simulink model "DQGEN"  (R2023b)
settings: Solver=ode23tb  StartTime=0.0  StopTime=0.1  FixedStep=Ts  RelTol=1e-5  EnableMultiTasking=on
values from neighbouring files (symbols this model uses):
  N = 2    [DQGEN_calc.m]
  Ts = 50e-6    (= 5e-05)    [DQGEN_calc.m]
  Ts_dqn = Ts    (= 5e-05)    [DQGEN_calc.m]
  Ws = 2*pi*f    (= 376.991118431)    [DQGEN_calc.m]
undefined symbols (not defined in the file or in its folder): DiscIntNeverNeededParam, rlc, SYS
libraries: spsThreePhaseVIMeasurementLib x3, DQN_Lib x2, spsLoadFlowBusLib x2, spsMultimeterLib x2, spsSteamTurbineandGovernorLib x2, spsThreePhaseSourceLib x1, spsGroundLib x1, spsSynchronousMachinepuStandardLib x1, spsThreePhaseParallelRLCBranchLib x1, spsThreePhaseSeriesRLCBranchLib x1, spsabctodq0Lib x1, spspowerguiLib x1
(part 1 of 2)
settings Model: NumberOfSteps=10  PacingRate=0.005000  Creator=The MathWorks, Inc.  LastModifiedBy=rober
settings SolverCC: ZeroCrossControl=DisableAll  ZeroCrossAlgorithm=Adaptive  AlgebraicLoopSolver=TrustRegion
settings DataIOCC: SaveFormat=Array  SaveOutput=off  SaveTime=off  ReturnWorkspaceOutputs=off  TimeSaveName=t  SignalLoggingName=sigsOut
settings OptimizationCC: BlockReduction=off  BooleanDataType=off  ExpressionDepthLimit=2147483647  InitFltsAndDblsToZero=on  EfficientMapNaN2IntZero=off  LifeSpan=inf
settings DebuggingCC: UnderspecifiedInitializationDetection=Classic  MergeDetectMultiDrivingBlocksExec=none  CheckExecutionContextPreStartOutputMsg=on  SignalResolutionControl=TryResolveAllWithWarning  IgnoredZcDiagnostic=none  MultiTaskDSMMsg=warning  MultiTaskCondExecSysMsg=none  FcnCallInpInsideContextMsg=warning  StateNameClashWarn=warning  SFUnexpectedBacktrackingDiag=warning  SFNoUnconditionalDefaultTransitionDiag=warning  SFExecutionAtInitializationDiag=none  ArithmeticOperatorsInVariantConditions=warning
settings HardwareCC: ProdBitPerPointer=32  ProdBitPerSizeT=32  ProdBitPerPtrDiffT=32  ProdLargestAtomicFloat=None  ProdIntDivRoundTo=Undefined  ProdEndianess=Unspecified  ProdWordSize=32  ProdHWDeviceType=32-bit Generic  TargetBitPerPointer=64  TargetBitPerSizeT=64  TargetBitPerPtrDiffT=64  TargetLongLongMode=on  TargetIntDivRoundTo=Zero  TargetEndianess=LittleEndian  TargetWordSize=64  TargetHWDeviceType=MATLAB Host  ProdEqTarget=off
settings ModelReferenceCC: EnableRefExpFcnMdlSchedulingChecks=on  PropagateSignalLabelsOutOfModel=off
settings SFSimCC: SimUseLocalCustomCode=off  CustomCodeUndefinedFunction=UseInterfaceOnly
settings RTWCC: RTWUseLocalCustomCode=off  DLArmComputeVersion=19.05
settings CodeAppCC: StateflowObjectComments=on
settings GRTTargetCC: TargetLangStandard=C89/C90 (ANSI)  CombineOutputUpdateFcns=off  GRTInterface=on
settings ConfigComp: CovMetricSettings=dw  CovSaveCumulativeToWorkspaceVar=on  CovSaveSingleToWorkspaceVar=on  CovExternalEMLEnable=off  CovSFcnEnable=off
settings SimscapeCC: SimscapeNormalizeSystem=off

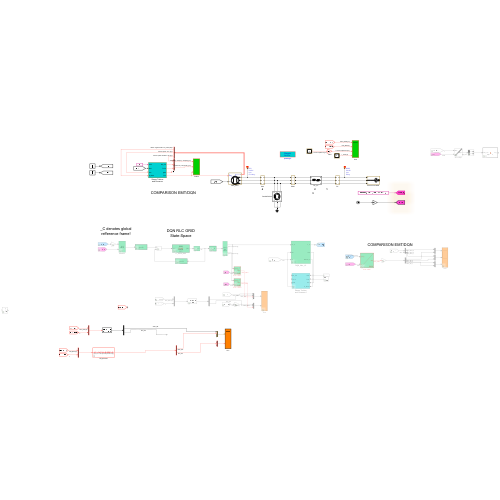
[thumbnail: Simulink's stored preview of the top-level diagram]
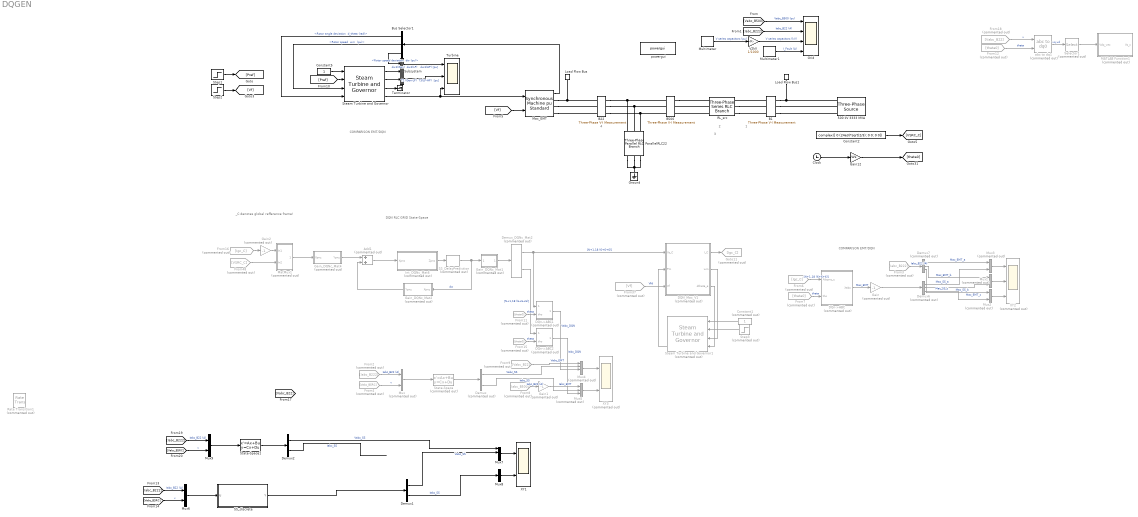
== system DQGEN ==
  note: DQN RLC GRID
      | State-Space
  note: 1
  note: 2
  note: 3
  note: 4
  note: COMPARISON EMT/DQN
  note: _C denotes global
      | refference frame!
  note: COMPARISON EMT/DQN
  500 kV 3333 MVA : spsThreePhaseSourceLib/Three-Phase Source  InternalConnection=Yg  VoltagePhases=off  Voltage=(24000)*1  PhaseAngle=0  Voltage_phases=[25e3 25e3 25e3]/sqrt(3)  PhaseAngles_phases=[0 -120 +120]  Frequency=60  NonIdealSource=off  SpecifyImpedance=on  Resistance=3.5  Inductance=0.1989  ShortCircuitLevel=3333e6  BaseVoltage=500e3  XRratio=21.43  BusType=swing  Pref=0  Qref=0  Prefabc=[10e3, 10e3, 10e3]  Qrefabc=[0, 0, 0]  Qmin=-Inf  Qmax=Inf
  Add1 : Sum  Commented=on
  B1 : spsThreePhaseVIMeasurementLib/Three-Phase V-I Measurement  VoltageMeasurement=phase-to-ground  SetLabelV=on  LabelV=Vabc_BSRC  Vpu=off  VpuLL=off  CurrentMeasurement=yes  SetLabelI=on  LabelI=Iabc_BSRC  Ipu=off  Pbase=100e6  Vbase=500e3  OutputType=Complex  PhasorSimulation=off  PSBequivalent=0
  B22 : spsThreePhaseVIMeasurementLib/Three-Phase V-I Measurement  VoltageMeasurement=phase-to-ground  SetLabelV=on  LabelV=Vabc_B22  Vpu=off  VpuLL=off  CurrentMeasurement=yes  SetLabelI=on  LabelI=Iabc_B222  Ipu=off  Pbase=555e6  Vbase=24e3  OutputType=Complex  PhasorSimulation=off  PSBequivalent=0
  B500 : spsThreePhaseVIMeasurementLib/Three-Phase V-I Measurement  VoltageMeasurement=phase-to-ground  SetLabelV=on  LabelV=Vabc_B500  Vpu=off  VpuLL=off  CurrentMeasurement=yes  SetLabelI=on  LabelI=Iabc_B500  Ipu=off  Pbase=100e6  Vbase=500e3  OutputType=Complex  PhasorSimulation=off  PSBequivalent=0
  Bus Selector1 : BusSelector  OutputSignals="Mechanical.Rotor angle deviation  d_theta (rad),Mechanical.Rotor speed  wm  (pu),Mechanical.Rotor speed deviation  dw (pu)"
  Clock : Clock
  Constant1 : Constant  Commented=on
  Constant2 : Constant  Value=complex([ 0 (24e3)*sqrt(2/3); 0 0; 0 0])
  Constant5 : Constant
  DQN_Mac_V1 : Subsystem  Commented=on  mask{HRM=N, NomParam=[ 555e6  24e3   60 ], reactVec=[1.81, 0.3, 0.23, 1.76, 0.65, 0.25, 0.15], timeConstVec=[ 1.3201, 0.0231, 0.3371, 0.0295 ], Rs=3.10E-03, Mech=[ 0.8788  0 1 ], lfVec=[0.9000   -0.0895    1.0000    1.8333    0.3334], Ts=Ts}
      mask prompts: HRM "Harmonic order:"; NomParam "Nominal power, line-to-line voltage, frequency [ Pn(VA)  Vn(Vrms)  fn(Hz) ]:"; reactVec "Reactances [ Xd  Xd'  Xd''  Xq  (Xq')  Xq''  Xl ] (pu):"; timeConstVec "[ Td'  Td''  (Tq')  Tq'' ] (s):"; Rs "Stator resistance Rs (pu):"; Mech "Inertia coefficient, friction factor, pole pairs [ H(s)  F(pu)  p()]:"; lfVec "Initial condition (phi(1x6), tho, dw) [1x8]:"; Ts "Integration timestep (s):"
      mask init:
      | SMRD = struct();
      | 
      |     SMRD.dwo = 0;
      | 
      |     SMRD.nState = numel(reactVec)-1;
      |     
      |     if(SMRD.nState>5)
      |         SMRD.RLinv   = zeros(6,6);
      |         SMRD.Linv    = zeros(6,6);
      |         SMRD.L       = zeros(6,6);
      |         SMRD.R       = zeros(6,6);
      |         W = zeros(6,6);
      |     else
      |         SMRD.RLinv   = zeros(5,5);
      |         SMRD.Linv    = zeros(5,5);
      |         SMRD.L       = zeros(5,5);
      |         SMRD.R       = zeros(5,5);
      |         W            = zeros(5,5);
      |     end
      | 
      |     SMRD.Rs      = Rs;
      | 
      |     SMRD.N       = 1;
      |     
      |     SMRD.H       = Mech(1);
      |     SMRD.F       = Mech(2);
      |     SMRD.p       = Mech(3);
      | 
      |     SMRD.Pn = NomParam(1);
      |     SMRD.Vn = NomParam(2);
      |     SMRD.fn = NomParam(3);
      |     
      |     
      |     Vb = SMRD.Vn*sqrt(2/3);
      |     Ib = sqrt(2/3)*SMRD.Pn/SMRD.Vn;
      |     
      |     
      |     Td_p    = timeConstVec(1);
      |     Td_pp   = timeConstVec(2);
      |     if(SMRD.nState>5)
      |         Tq_p    = timeConstVec(3);
      |         Tq_pp   = timeConstVec(4);
      |     else
      |         Tq_pp   = timeConstVec(3);
      |     end
      |     
      |     
      |     %Set the time constants in Lq(s)
      |     %See (eq. 7.2.14)
      |     
      |     wn=2*pi*SMRD.fn;
      |     SMRD.wn = wn;%Rated frequency in rad/sec
      |     %Implementation of the formulas in 
      |     
      |     % Xaq=1.165; %Mutual inductance
      |     % Ll=.188; %Stator leakage inductance
      |     
      |     %T5=0.0234;
      |     
      |     
      |     Xd      = reactVec(1);
      |     Xd_p    = reactVec(2);
      |     Xd_pp   = reactVec(3);
      |     Xq      = reactVec(4);
      | 
      | 
      |     if(SMRD.nState>5)
      |         Xq_p    = reactVec(5);
      |         Xq_pp   = reactVec(6);
      |         Xl      = reactVec(7);
      | 
      |         Tqo_p   = Tq_p * Xq/Xq_p;
      |         Tqo_pp  = Tq_pp * Xq_p/Xq_pp;
      |     else
      |         Xq_pp   = reactVec(5);
      |         Xl      = reactVec(6);
      |         Tqo_pp  = Tq_pp * Xq/Xq_pp;
      |     end
      | 
      | 
      |     Xad     = Xd-Xl; %Mutual inductance
      |     Xaq     = Xq-Xl; %Mutual inductance
      |     
      |     
      |     SMRD.Xd = Xd;
      |     SMRD.Xq = Xq;
      |     SMRD.Xl = Xl;
      |     SMRD.Xad = Xad;
      |     SMRD.Xaq = Xaq;
      |     
      |         
      |    
      |     LAM1 = sqrt(Xd^2*Xd_pp^2*(Td_p-Td_pp)^2+2*Td_p*Td_pp*Xd*Xd_p*Xd_pp*(Xd-2*Xd_p+Xd_pp)-2*Td_pp*Xd*Xd_p*Xd_pp*(Xd-Xd_p+Xd_pp)+Td_pp^2*Xd_pp^2*(Xd^2+Xd_pp^2));
      |     Tdo_p  = (Td_p*Xd*Xd_pp+LAM1+Td_pp*(Xd*Xd_p+Xd_p*Xd_pp-Xd*Xd_pp))/(2*Xd_p*Xd_pp);
      |     Tdo_pp = Xd*Td_p*Td_pp/(Xd_pp*Tdo_p);
      |     % 
      |     % Tqo_p   = Tq_p * Xq/Xq_p;
      |     % Tqo_pp  = Tq_pp * Xq_p/Xq_pp;
      |     
      |    
      |     %%%%%%%%%%%%%%%%%%%%%%
      |         
      |     a=SMRD.Xad*(Xd_p-SMRD.Xl)/(Xd-Xd_p);
      |     b=a*SMRD.Xad*(Xd_pp-SMRD.Xl)/(a*Xd+SMRD.Xl*SMRD.Xad-(a+SMRD.Xad)*Xd_pp);
      |     c=(b+a*SMRD.Xl*SMRD.Xad/(SMRD.Xl*SMRD.Xad+a*Xd))/Td_pp;
      |     
      |     T5 = b/c;
      |     
      |     %%%%%%%%%%%%%%%%%%%%%%%%% D AXIS %%%%%%%%%%%%%%%%%%%%%%%%%
      |     
      |     SMRD.Ro=SMRD.wn*Xd*(Tdo_p+Tdo_pp-Td_p-Td_pp);
      |     SMRD.Ro=SMRD.Xad*SMRD.Xad/SMRD.Ro;
      |     
      |     
      |     a=Xd*(Td_p+Td_pp)-SMRD.Xl*(Tdo_p+Tdo_pp);a=a/SMRD.Xad;
      |     b=Xd*Td_p*Td_pp-SMRD.Xl*Tdo_p*Tdo_pp; b=b/SMRD.Xad;
      |     c=(Tdo_p*Tdo_pp-Td_p*Td_pp)/(Tdo_p+Tdo_pp-Td_p-Td_pp);
      |     
      |     % T5=0.0234;
      |     
      |     SMRD.Lf1d=b-a*T5+T5*T5; %in p.u.
      |     SMRD.Lf1d=SMRD.Ro*SMRD.Lf1d/(c-T5); %in p.u.
      |     SMRD.Rfd=SMRD.Ro*(SMRD.Lf1d+SMRD.Ro*(2*T5-a)); 
      |     SMRD.Rfd=SMRD.Rfd/(SMRD.Lf1d+SMRD.Ro*(T5+c-a));%in p.u.
      |     SMRD.Lfd=SMRD.Rfd*(a-T5-SMRD.Lf1d/SMRD.Ro); %in p.u.
      |     SMRD.R1d=SMRD.Ro*SMRD.Rfd/(SMRD.Rfd-SMRD.Ro); %in p.u. 
      |     %Inductances in p.u.
      |     SMRD.L1d=SMRD.R1d*T5; SMRD.L1d=SMRD.L1d*SMRD.wn; 
      |     SMRD.Lfd=SMRD.Lfd*SMRD.wn; SMRD.Lf1d=SMRD.Lf1d*SMRD.wn;
      |     
      |     %%%%%%%%%%%%%%%%%%%%%%%%%%%%%%%%%%%%%%%%%%%%%%%%%%%%%%%%%%
      |     
      |     %%%%%%%%%%%%%%%%%%%%%%%%% Q AXIS %%%%%%%%%%%%%%%%%%%%%%%%% Tqo′ Xq″ Xq SMRD.Xl 
      |     
      |     if(SMRD.nState>5)
      |         %conv(x,y)= polynomial multiplication
      |         N=conv([Tq_p 1],[Tq_pp 1]); 
      |         D=conv([Tqo_p 1],[Tqo_pp 1]);
      |         Nz=conv(N-D*SMRD.Xl/Xq,[Xaq/SMRD.wn 0]);
      |         Dz=D-N; Nz=Nz(1:3); Dz=Dz(1:2);
      |         Req=Nz(3)/Dz(2);
      |         Nz=Nz/Nz(3); Dz=Dz/Dz(2);
      |         %compute polynomial roots and sort them
      |         Tab=sort(abs(roots(Nz))); Tab=1./Tab;
      |         Tm=sort(abs(roots(Dz))); Tm=1/Tm(1);
      |         %Solve a system of two linear equa�tions
      |         x=[1 1;Tab(1) Tab(2)]\[1 ;Tm]/Req;
      |         %Results
      |         SMRD.R1q=1/x(1); 
      |         SMRD.L1q=SMRD.wn*SMRD.R1q*Tab(1); %in p.u.
      |         SMRD.R2q=1/x(2); 
      |         SMRD.L2q=SMRD.wn*SMRD.R2q*Tab(2); %in p.u.
      |     else
      |         N=conv([1],[Tq_pp 1]); 
      |         D=conv([1],[Tqo_pp 1]);
      |         Nz=conv(N-D*SMRD.Xl/Xq,[Xaq/SMRD.wn 0]);
      |         Dz=D-N; Nz=Nz(1:2); Dz=Dz(1:1);
      |         Req=Nz(2)/Dz(1);
      |         Nz=Nz/Nz(2); Dz=Dz/Dz(1);
      |         %compute polynomial roots and sort them
      |         Tab=sort(abs(roots(Nz))); Tab=1./Tab;
      |         Tm=1;
      |         %Solve a system of two linear equa�tions
      |         x=[1;Tab(1)]/Req;
      |         %Results
      |         SMRD.R1q=1/x(1); 
      |         SMRD.L1q=SMRD.wn*SMRD.R1q*Tab(1); %in p.u.
      |     end
      |     
      |     %%%%%%%%%%%%%%%%%%%%%%%%%%%%%%%%%%%%%%%%%%%%%%%%%%%%%%%%%%
      |     
      |     
      |     if(1)
      |         T11d = T5;
      |         
      |         K1 = (Tdo_p+Tdo_pp-Td_p-Td_pp)*(Tdo_p*Tdo_pp*(Td_p+Td_pp)-Td_p*Td_pp*(Tdo_p+Tdo_pp))-(Tdo_p*Tdo_pp-Td_p*Td_pp)^2;    
      |         
      |         
      |         %K2 = Rfd*K1*Ld/(Lad^2);
      |         K2 = (Tdo_p*Tdo_pp*(Td_p+Td_pp)-Td_p*Td_pp*(Tdo_p+Tdo_pp)+T11d^2*(Tdo_p+Tdo_pp-Td_p-Td_pp)-2*T11d*(Tdo_p*Tdo_pp-Td_p*Td_pp))/SMRD.wn;
      |         K3 = Tdo_p*Tdo_pp-T11d*(Tdo_p+Tdo_pp-T11d);
      |         K4 = Tdo_p*Tdo_pp-Td_p*Td_pp-T11d*(Tdo_p+Tdo_pp-Td_p-Td_pp);
      |         K5 = Tdo_p*Tdo_pp*(Td_p+Td_pp)-Td_p*Td_pp*(Tdo_p+Tdo_pp)-T11d*(Tdo_p*Tdo_pp-Td_p*Td_pp);
      |         
      |         Rfd_R = Xad^2*K2/(Xd*K1);
      |         
      |         Lf1d_R = (Xad^2*K3/(Xd*K4)-Xad)*wn; %Lf1d
      |         Lfd_R = Rfd_R*K5/K4*wn; %Lfd
      |         R1d_R = Rfd_R*K1/K4^2;
      |         L1d_R = Rfd_R*T5*wn;
      |         
      |         SMRD.Rfd_R  = Rfd_R;
      |         SMRD.Lf1d_R = Lf1d_R;
      |         SMRD.Lfd_R = Lfd_R;
      |         SMRD.R1d_R = R1d_R;
      |         SMRD.L1d_R = L1d_R;
      |     end
      |     
      | 
      |     %%%%%%%%%%%%%%%%%%%%%%%%% R/L MAT %%%%%%%%%%%%%%%%%%%%%%%%%
      | 
      |     Ro=Xad*Xad/(wn*Xd*(Tdo_p+Tdo_pp-Td_p-Td_pp));
      | 
      |     if(SMRD.nState>5)
      |         SMRD.L(1,1) = SMRD.Xd; SMRD.L(1,3) = SMRD.Xad; SMRD.L(1,5) = SMRD.Xad;
      |         SMRD.L(2,2) = SMRD.Xq; SMRD.L(2,4) = SMRD.Xaq; SMRD.L(2,6) = SMRD.Xaq;
      |         SMRD.L(3,1) = SMRD.Xad; SMRD.L(3,3) = SMRD.Xad + SMRD.Lf1d + SMRD.L1d; SMRD.L(3,5) = SMRD.Lf1d + SMRD.Xad;
      |         SMRD.L(4,2) = SMRD.Xaq; SMRD.L(4,4) = SMRD.Xaq + SMRD.L1q; SMRD.L(4,6) = SMRD.Xaq;
      |         SMRD.L(5,1) = SMRD.Xad; SMRD.L(5,3) = SMRD.Xad + SMRD.Lf1d; SMRD.L(5,5) = SMRD.Lf1d + SMRD.Xad + SMRD.Lfd;
      |         SMRD.L(6,2) = SMRD.Xaq; SMRD.L(6,4) = SMRD.Xaq; SMRD.L(6,6) = SMRD.Xaq + SMRD.L2q;
      |     else
      |         SMRD.L(1,1) = SMRD.Xd; SMRD.L(1,3) = SMRD.Xad; SMRD.L(1,5) = SMRD.Xad;
      |         SMRD.L(2,2) = SMRD.Xq; SMRD.L(2,4) = SMRD.Xaq; %SMRD.L(2,6) = SMRD.Xaq;
      |         SMRD.L(3,1) = SMRD.Xad; SMRD.L(3,3) = SMRD.Xad + SMRD.Lf1d + SMRD.L1d; SMRD.L(3,5) = SMRD.Lf1d + SMRD.Xad;
      |         SMRD.L(4,2) = SMRD.Xaq; SMRD.L(4,4) = SMRD.Xaq + SMRD.L1q; %SMRD.L(4,6) = SMRD.Xaq;
      |         SMRD.L(5,1) = SMRD.Xad; SMRD.L(5,3) = SMRD.Xad + SMRD.Lf1d; SMRD.L(5,5) = SMRD.Lf1d + SMRD.Xad + SMRD.Lfd;
      |         %SMRD.L(6,2) = SMRD.Xaq; SMRD.L(6,4) = SMRD.Xaq; SMRD.L(6,6) = SMRD.Xaq + SMRD.L2q;
      |     end
      |     
      |     
      | 
      |     
      |     W(2,1) = +1;
      |     W(1,2) = -1;
      |     
      |    if(SMRD.nState>5) 
      |     SMRD.R(1,1) = Rs;
      |     SMRD.R(2,2) = Rs;
      |     SMRD.R(3,3) = Rfd_R;
      |     SMRD.R(4,4) = SMRD.R1q;
      |     SMRD.R(5,5) = R1d_R;
      |     SMRD.R(6,6) = SMRD.R2q;
      |    else
      |     SMRD.R(1,1) = Rs;
      |     SMRD.R(2,2) = Rs;
      |     SMRD.R(3,3) = Rfd_R;
      |     SMRD.R(4,4) = SMRD.R1q;
      |     SMRD.R(5,5) = R1d_R;
      |    end
      |     
      |     %%%%%%%%%%%%%%%%%%%%%%%%%%%%%%%%%%%%%%%%%%%%%%%%%%%%%%%%%%
      |     
      |     
      |     a=(Xd*(Td_p+Td_pp)-Xl*(Tdo_p+Tdo_pp))/Xad;
      |     b=(Xd*Td_p*Td_pp-Xl*Tdo_p*Tdo_pp)/Xad;
      |     c=(Tdo_p*Tdo_pp-Td_p*Td_pp)/(Tdo_p+Tdo_pp-Td_p-Td_pp);
      |     Lf1d=b-a*T5+T5*T5; %in p.u.
      |     Lf1d=Ro*Lf1d/(c-T5); %in p.u.
      |     %Rfd=Ro*(Lf1d+Ro*(2*T5-a));
      |     Rfd=Ro*(Lf1d+Ro*(2*T5-a))/(Lf1d+Ro*(T5+c-a));%in p.u.
      |     Lfd=Rfd*(a-T5-Lf1d/Ro); %in p.u.
      |     R1d=Ro*Rfd/(Rfd-Ro); %in p.u.
      |     %Inductances in p.u.
      |     L1d=R1d*T5; 
      |     L1d=L1d*wn;
      |     Lfd=Lfd*wn; 
      |     Lf1d=Lf1d*wn;
      |      
      |     
      |     a = Xad*(Xd_p-Xl)/(Xd-Xd_p);
      |     b = Xad*(Xd_pp-Xl)/(a*Xd+Xl*Xad-(a+Xad)*Xd_pp);
      |     c = (1/Td_pp)*(b- (a*Xl*Xad)/(Xl*Xad+a*Xd) );
      |     
      |     T11d = b/c;
      |     
      |     
      |     Xf1d = Xad^2*K3/(Xd*K4)-Xad;
      |     X1d = T11d*Rfd - K1/K4^2;
      |     
      |     SMRD.Xf1d = Xf1d;
      |     SMRD.X1d = X1d;
      |     
      |     %%%%%%%%%%%%%%%%%%%%%%%%%%%%% LF  %%%%%%%%%%%%%%%%%%%%%%%%%
      |     
      |     Pt = lfVec(1);
      |     Qt = lfVec(2);
      |     Vt = lfVec(3);
      |     Et = lfVec(4);
      |     At = lfVec(5);
      |     % if(numel(lfVec)>5) fac = lfVec(6); end
      |     
      |     phi = At;
      |     
      |     It = sqrt(Pt^2+Qt^2)/Vt; 
      |     
      |     Xd = reactVec(1);
      |     Xq = reactVec(4);
      | 
      |     Xmd = Xd-Xl;
      |     
      |     fi = sign(Qt)*acos(Pt/(Vt*It)); rad2deg(fi)
      |     
      |     del = (atan((Xq*It*cos(fi)-Rs*It*sin(fi))/(Vt+Rs*It*cos(fi)+Xq*It*sin(fi))));
      |     
      |     SMRD.del = del;
      |     
      |     tho = del+phi-pi/2;
      |     
      |     SMRD.Vfnp = ((Rfd*Vb/(Xmd*wn))^2);
      |     
      |     v_dq = Vt*exp(1i*(pi/2-del)); %correct
      |     ed = real(v_dq);
      |     eq = imag(v_dq);
      |     efd = Et*SMRD.Vfnp;
      |     
      |     
      |     v_vec = [ed; eq; efd; zeros(SMRD.nState-3,1)];
      |     i_vec = (v_vec'/(SMRD.R-SMRD.L*W))';
      | 
      |     %%%%%%%%%%%%%%%%%%%%%%%%%%%%%%%%%%%%%%%%%%%%%%%%%%%%%%%%%%
      |     
      |     SMRD.idq0 = i_vec;
      |     SMRD.phidq0 = SMRD.L*i_vec;
      |     SMRD.tho = tho;
      |     SMRD.dwo = 0;
      | 
      |     SMRD.Linv = eye(SMRD.nState)/SMRD.L;
      |     SMRD.RLinv = SMRD.R*SMRD.Linv;
      | 
      | 
      |     SMRD.Pb = 1;
      |     SMRD.Ib = Ib;
      |     SMRD.Vb = Vb;
      | 
      |     SMRD.IqdSign = [-1    -1     ones(1,SMRD.nState-2)];
      | 
      |     SMRD.Vt = Vt*exp(1i*(phi));
      |     SMRD.It = (Pt-1i*Qt)/(Vt*exp(-1i*(phi)));
      |     SMRD.Ts = Ts;
      |     SMRD.web = SMRD.wn;
      settings: LibrarySourceBlock=|
      | spsSynchronousMachineModel/Continuous/Synchronous Machine
      | Continuous Model
  DQn->ABC : MATLAB Function  Commented=on  TreatAsAtomicUnit=on  SystemSampleTime=Ts  mask{N=N}
      mask prompts: N "Harmonic order:"
  DQn->ABC1 : MATLAB Function  Commented=on  TreatAsAtomicUnit=on  SystemSampleTime=Ts  mask{N=N}
      mask prompts: N "Harmonic order:"
  DQn->ABC2 : MATLAB Function  Commented=on  TreatAsAtomicUnit=on  SystemSampleTime=Ts  mask{N=N}
      mask prompts: N "Harmonic order:"
  Demux : Demux  Commented=on  Outputs=2
  Demux1 : Demux  Outputs=2
  Demux2 : Demux  Outputs=2
  Demux6 : Demux  Commented=on  Outputs=3
  Demux7 : Demux  Commented=on  Outputs=3
  Demux_DQNc_Mat2 : DQN_Lib/Demux_DQNc_Mat  Commented=on  nrOut=2
  From{7,11..12,15} (4 alike) : From  Commented=on  GotoTag=theta0
  From16 : From  Commented=on  GotoTag=Igc_C
  From18 : From  Commented=on  GotoTag=Vabc_B22  TagVisibility=global
  From2 : From  Commented=on  GotoTag=Iabc_B222  TagVisibility=global
  From3 : From  Commented=on  GotoTag=Iabc_B222  TagVisibility=global
  From37 : From  Commented=on  GotoTag=Vf
  From4 : From  Commented=on  GotoTag=Vabc_BSRC  TagVisibility=global
  From48 : From  Commented=on  GotoTag=VSRC_C
  From6 : From  Commented=on  GotoTag=Igc_C
  From8 : From  Commented=on  GotoTag=Iabc_B500  TagVisibility=global
  From9 : From  Commented=on  GotoTag=Vabc_B22  TagVisibility=global
  Gain : Gain  Commented=on  Gain=-1
  Gain1 : Gain  Commented=on  Gain=-1
  Gain12 : Gain  Gain=Ws
  Gain2 : Gain  Commented=on  Gain=-1
  Gain_DQNc_Mat1 : MATLAB Function  Commented=on  TreatAsAtomicUnit=on  SystemSampleTime=Ts  mask{Rabc=SYS.C, HRM=N, chkInv=off}
      mask prompts: Rabc "Line matrix [3x3]:"; HRM "Harmonic order:"; chkInv "Invert"
  Gain_DQNc_Mat2 : MATLAB Function  Commented=on  TreatAsAtomicUnit=on  SystemSampleTime=Ts  mask{Rabc=SYS.A, HRM=N, chkInv=off}
      mask prompts: Rabc "Line matrix [3x3]:"; HRM "Harmonic order:"; chkInv "Invert"
  Gain_DQNc_Mat4 : MATLAB Function  Commented=on  TreatAsAtomicUnit=on  SystemSampleTime=Ts  mask{Rabc=SYS.B, HRM=N, chkInv=off}
      mask prompts: Rabc "Line matrix [3x3]:"; HRM "Harmonic order:"; chkInv "Invert"
  Goto11 : Goto  Commented=on  GotoTag=Igc_C
  Grid : Scope  NumInputPorts=4
  Ground : spsGroundLib/Ground  LConnTagsString=a
  Int_DQNc_Mat6 : MATLAB Function  Commented=on  TreatAsAtomicUnit=on  mask{N=N, dt=Ts_dqn, w=Ws, InitInt=SYS.x0, swFeed=off, R=-SYS.A, iL=eye(size(SYS.A,1))}
      mask prompts: N "Order number:"; dt "Time step (s):"; w "Angular frequency (1/rad):"; InitInt "Initial conditions DC [3x1]:"; swFeed "Enable feedback"; R "Feedback parameter (Kr {abc}):"; iL "Feedback parameter (Ki {abc}):"
  Load Flow Bus : spsLoadFlowBusLib/Load Flow Bus  LConnTagsString=a  Phases=single  Connectors=on one side  ID=B22  Vbase=24e3  Vref=1  Vangle=0  VLF=1  VLFb=1  VLFc=1  angleLF=19.1  angleLFb=0  angleLFc=0
      settings: AttributesFormatString=%<ID>\n%<Vbase>V\n%<VLF>pu\n%<angleLF>deg.
  Load Flow Bus1 : spsLoadFlowBusLib/Load Flow Bus  LConnTagsString=a  Phases=single  Connectors=on one side  ID=BSRC  Vbase=24e3  Vref=1  Vangle=0  VLF=1  VLFb=1  VLFc=1  angleLF=0  angleLFb=0  angleLFc=0
      settings: AttributesFormatString=%<ID>\n%<Vbase>V\n%<VLF>pu\n%<angleLF>deg.
  MATLAB Function1 : MATLAB Function  Commented=on  TreatAsAtomicUnit=on  mask{N=N}
      mask prompts: N "Harmonic order:"
  Mac_EMT : spsSynchronousMachinepuStandardLib/Synchronous Machine pu Standard  PresetModel=No  MechanicalLoad=Mechanical power Pm  ShowDetailedParameters=on  RotorType=Round  Units=per unit standard parameters  MeasurementBus=off  NominalParameters="[ 555e6  24e3   60 ]"  Reactances1=[1.81, 0.3, 0.23, 1.76, 0.65, 0.25, 0.15]  Reactances2="[ 1.305, 0.296, 0.252, 0.474,  0.243,  0.18 ]"  dAxisTimeConstants=Short-circuit  qAxisTimeConstants=Short-circuit  TimeConstants1="[ 4.4849  0.0681  0.1  ]"  TimeConstants2=[8, 0.03, 1, 0.07]  TimeConstants3="[  4.49  0.0681  0.0513  ]"  TimeConstants4=[ 8.0, 0.03, 0.3371, 0.0295 ]  TimeConstants5=[ 1.01, 0.053, 0.1 ]  TimeConstants6=[ 1.3201, 0.023, 1.0, 0.07 ]  TimeConstants7="[  1.01  0.053  0.051266  ]"  TimeConstants8=[ 1.3201, 0.0231, 0.3371, 0.0295 ]  StatorResistance=3.10E-03  Mechanical="[ 0.8788  0 1 ]"  PolePairs=1  InitialConditions=[0 -8.98302 0.904437 0.904437 0.904437 24.7773 -95.2227 144.777 1.83328]  SetSaturation=off  Saturation=[0.6404,0.7127,0.8441,0.9214,0.9956,1.082,1.19,1.316,1.457;0.7,0.7698,0.8872,0.9466,0.9969,1.046,1.1,1.151,1.201]  LoadFlowParameters=[1 0 0 0 0]  TsPowergui=0  TsBlock=Ts  IterativeModel=Trapezoidal non iterative  IterativeDiscreteModel=Trapezoidal robust  BusType=PV  Pref=499500000  Qref=-222000000  Qmin=-Inf  Qmax=Inf  PLF=0  QLF=0
  MatMux1 : Subsystem  Commented=on  mask{nrInp=2}
      mask prompts: nrInp "Number of inputs [{C}]"
      mask init:
      | %blocks = find_system(gcb,'LookUnderMasks','on','FollowLinks','on')
      | %set_param(gcb, 'MaskSelfModifiable', 'on');
      | 
      | % if(SSM == [])
      | %     Simulink.SubSystem.deleteContents(gcb);
      | % else
      | 
      | if(isempty(nrInp))
      |     Simulink.SubSystem.deleteContents(gcb);
      | else
      | 
      |     nrOut = 1;
      | 
      | 
      | PortHandles = get_param(gcb,'PortHandles');
      | lenInp = length(PortHandles.Inport);
      | lenOut = length(PortHandles.Inport);
      | 
      | if(nrInp ~= lenInp)
      |     %disp('ENTERED')
      |     Simulink.SubSystem.deleteContents(gcb);
      | %     add_block('simulink/Continuous/State-Space', [gcb,'/ss_block'], 'A','SS.A', 'B','SS.B', 'C','SS.C', 'D','SS.D', 'X0','X0')
      | %     set_param([gcb,'/ss_block'],'position' , [350,100,450,150])
      | 
      | 
      | 
      |         add_block('simulink/Math Operations/Matrix Concatenate',[gcb,'/Mux'], 'NumInputs',num2str(nrInp), 'ConcatenateDimension',num2str(2));
      |         set_param([gcb,'/Mux'],'position' , [200,100,250,100+nrInp*50])
      |         
      | %         add_block('built-in/Demux',[gcb,'/Demux'], 'Outputs',num2str(nrOut));
      | %         set_param([gcb,'/Demux'],'position' , [500,100,550,100+nrOut*50])
      | 
      | 
      |         for i = 1 : nrInp
      |             add_block('built-in/Inport',[gcb,strcat('/In',num2str(i))]);
      |             set_param([gcb,strcat('/In',num2str(i))],'position' , [50,65+i*50,90,85+i*50]);
      |             add_line(gcb,strcat('In',num2str(i),'/1'),strcat('Mux/',num2str(i)),'autorouting','on');
      |         end
      | 
      |         for i = 1 : nrOut
      |             add_block('built-in/Outport',[gcb,strcat('/Out',num2str(i))]);
      |             set_param([gcb,strcat('/Out',num2str(i))],'position' , [750,65+i*50,790,85+i*50]);
      |             add_line(gcb,strcat('Mux/',num2str(i)), strcat('Out',num2str(i),'/1'),'autorouting','on');
      |         end
      | 
      | 
      | %     add_line(gcb, 'Mux/1', 'ss_block/1')
      | %     add_line(gcb, 'ss_block/1', 'Demux/1')
      | 
      | end
      | 
      | end
      mask Display: disp(['{\color{red}\bf\fontsize{12}} [\{C\}]',newline,' MUX'], 'texmode','on');
  Multimeter : spsMultimeterLib/Multimeter  L=6  sel=[1 2 3]  yselected={}  Gain=[1 1 1]  OutputType=Complex  PlotAtSimulationStop=off  PhasorSimulation=off
  Multimeter1 : spsMultimeterLib/Multimeter  L=6  sel=1  yselected={}  Gain=0  OutputType=Complex  PlotAtSimulationStop=off  PhasorSimulation=off
  Mux{,1..3} (4 alike) : Mux  Commented=on  Inputs=2
  Mux4 : Mux  Commented=on
  Mux5 : Mux  Commented=on  Inputs=3
  Mux6 : Mux  Inputs=2
  Mux7 : Mux
  Mux8 : Mux  Inputs=3
  Mux9 : Mux  Inputs=2
  ParallelRLC22 : spsThreePhaseParallelRLCBranchLib/Three-Phase Parallel RLC Branch  LConnTagsString=A|B|C  RConnTagsString=A|B|C  BranchType=RC  Resistance=rlc(4,4)  Inductance=1e-3  Capacitance=rlc(4,6)*1e-6  Measurements=Branch voltages
  RL_src : spsThreePhaseSeriesRLCBranchLib/Three-Phase Series RLC Branch  LConnTagsString=A|B|C  RConnTagsString=A|B|C  BranchType=RL  Resistance=rlc(1,4)  Inductance=rlc(1,5)*1e-3  Capacitance=1/(0.55*0.080*(500e3^2/100e6))/(2*pi*60)  Measurements=Branch voltages
  Rate Transition1 : RateTransition  Commented=on  Deterministic=off  OutPortSampleTime=Ts
  SS_DelayPrediction : DQN_Lib/SS_DelayPrediction  Commented=on  N=N  Ts=Ts  x0=SYS.x0
  SS_discrete : Subsystem  mask{A=SYS.A, B=SYS.B, C=SYS.C, D=SYS.D, InitVec=SYS.x0, dt=Ts}
      mask prompts: InitVec "Initial condition:"; dt "Time step (s):"
      settings: LibrarySourceBlock=|
      | spsSynchronousMachineModel/Discrete robust/State Space Model/Discretize
      | BE or Tustin
      mask Display: disp(['{\color{red}\bf\fontsize{12}x(t) = Ad*x(t-dt)+Bd*u(t)}',newline,'{\color{gray}\bf\fontsize{12}y(t) = Cd*x(t-dt)+Dd*u(t)}'], 'texmode','on');
  Selector1 : Selector  Commented=on  InputPortWidth=3  IndexOptions=Index vector (dialog)  Indices=[1 2]  OutputSizes=1
  State-Space : StateSpace  Commented=on  A=SYS.A  B=SYS.B  C=SYS.C  D=SYS.D  InitialCondition=SYS.x0
  State-Space1 : StateSpace  A=SYS.A  B=SYS.B  C=SYS.C  D=SYS.D  InitialCondition=SYS.x0
  Steam Turbine and Governor : spsSteamTurbineandGovernorLib/Steam Turbine and Governor  gentype=Tandem-compound (multi-mass)  reg1="[ 1  0.05    0 ]"  reg2="[ 0.001  0.15 ]"  reg3="[ -0.1  0.1  0  4.496]"  N=3600  turb1="[ 0  10   3.3   0.5   ]"  turb2="[ 0.5   0.5   0  0 ]"  HA="[  1.5498   0.24894  0  0 ]"  KA="[  83.47  42.702  0  0 ]"  DA="[  0.3104  0.05  0  0 ]*8"  ini1=250.35/555  ini2=[0.90254 -8.983]
  Steam Turbine and Governor1 : spsSteamTurbineandGovernorLib/Steam Turbine and Governor  Commented=on  gentype=Tandem-compound (multi-mass)  reg1="[ 1  0.05    0 ]"  reg2="[ 0.001  0.15 ]"  reg3="[ -0.1  0.1  0  4.496]"  N=3600  turb1="[ 0  10   3.3   0.5   ]"  turb2="[ 0.5   0.5   0  0 ]"  HA="[  1.5498   0.24894  0  0 ]"  KA="[  83.47  42.702  0  0 ]"  DA="[  0.3104  0.05  0  0 ]*8"  ini1=250.35/555  ini2=[0.90254 -8.983]
  Step1 : Step  Time=5  Before=0.9  After=0.6  SampleTime=0
  Step2 : Step  Time=7  Before=1.8333  After=10  SampleTime=0
  Step3 : Step  Commented=on  Time=5  Before=0.9  After=0.6  SampleTime=0
  Subsystem : Subsystem
  Terminator : Terminator
  Turbine : Scope  NumInputPorts=3
  V2kV : Gain  Gain=1/1000
  XY1 : Scope  NumInputPorts=2
  XY2 : Scope  Commented=on  NumInputPorts=3
  XY3 : Scope  Commented=on  NumInputPorts=2
  abc to dq1 : spsabctodq0Lib/abc to dq0  Commented=on  Alignment=90 degrees behind phase A axis
  powergui : spspowerguiLib/powergui  Priority=2  SimulationMode=Discrete  SampleTime=Ts  frequency=60  Iterations=50  frequencyindice=60  Pbase=100e6  ErrMax=0.0001  UnitsV=kV  UnitsW=MW  buscounter=0  FunctionMessages=off  echomessages=off  EnableUseOfTLC=off  CurrentSourceSwitches=off  DisableSnubberDevices=off  DisableRonSwitches=off  DisableVfSwitches=off  DisplayEquations=off  AutomaticDiscreteSolvers=off  SolverType=Tustin/Backward Euler (TBE)  Interpol=off  ExternalGateDelay=off  methode=off  Ts=0  x0status=blocks  SPID=on  SwTol=0  HookPort=off  NonlinearTolerance=1e-4  nMaxIteration=100  ContinueOnMaxIteration=off  RestoreLinks=warning  ResistiveCurrentMeasurement=off  Frange=logspace(0,3,50)  Ylog=off  Xlog=off  ShowGrid=off  save=off  variable=ZData  structure=0  ZoomFFT=on  StartTime=0.0  cycles=2  DisplayStyle=off  fundamental=60  FreqAxis=off  MaxFrequency=1000  frequencyindicesteady=1  RmsSteady=1  display=off
  wires:
  [Vabc_B500] -> Grid/1  "Vabc_B500 (pu)"
  [Iabc_B222] -> Grid/2  "Iabc_B22 (A)"
  Multimeter/1 -> V2kV/1  "V series capacitors (pu)"
  V2kV/1 -> Grid/3  "V series capacitors (kV)"
  Multimeter1/1 -> Grid/4  "I_Fault (A)"
  Step2/1 -> [Vf]
  Steam Turbine and Governor/4 -> Turbine/3, Mac_EMT/1
  Steam Turbine and Governor/3 -> Terminator/1
  [Pref] -> Steam Turbine and Governor/2
  Bus Selector1/2 -> Steam Turbine and Governor/3  "<Rotor speed  wm  (pu)>"
  Subsystem/2(T_23) -> Turbine/2  "T2 (Gen-LP)  T3(LP-HP)  [pu]"
  Bus Selector1/3 -> Subsystem/1(In1)  "<Rotor speed deviation  dw (pu)>"
  Steam Turbine and Governor/1 -> Subsystem/2(In2)
  Mac_EMT/1 -> Bus Selector1/1
  Subsystem/1(dw_123) -> Turbine/1  "dw1(Gen)  dw2(LP)   dw3(HP) [pu]"
  Bus Selector1/1 -> Steam Turbine and Governor/4  "<Rotor angle deviation  d_theta (rad)>"
  Constant5/1 -> Steam Turbine and Governor/1
  Steam Turbine and Governor/2 -> Subsystem/3(In3)
  From6/1 -> DQn->ABC/1(Xdcpnz_c)  "[N+1,18 (6+6+6)]"
  Constant2/1 -> [VSRC_C]
  Int_DQNc_Mat6/1(Zpnz) -> SS_DelayPrediction/1
  MatMux1/1(Out1) -> Gain_DQNc_Mat4/1(Xpnz)
  SS_DelayPrediction/1 -> Gain_DQNc_Mat1/1(Xpnz), Gain_DQNc_Mat2/1(Xpnz)  "dw"
  Gain_DQNc_Mat4/1(Ypnz) -> Add1/1
  Add1/1 -> Int_DQNc_Mat6/1(Xpnz)
  Gain_DQNc_Mat2/1(Ypnz) -> Add1/2
  Gain_DQNc_Mat1/1(Ypnz) -> Demux_DQNc_Mat2/1
  DQN_Mac_V1/1(I_C) -> Goto11/1
  From48/1 -> MatMux1/2(In2)
  Demux6/2 -> Mux1/2  "Mac_SS_b"
  Demux7/2 -> Mux1/1  "Mac_EMT_b"
  DQn->ABC/1(Xabc) -> Gain/1  "Mac_EMT"
  Demux7/1 -> Mux3/1  "Mac_EMT_a"
  Mux1/1 -> XY2/2
  Mux3/1 -> XY2/1
  Demux7/3 -> Mux2/1  "Mac_EMT_c"
  Demux6/3 -> Mux2/2  "Mac_SS_c"
  Demux6/1 -> Mux3/2  "Mac_SS_a"
  From3/1 -> Demux7/1  "Iabc_B22 (A)"
  Mux2/1 -> XY2/3
  From37/1 -> DQN_Mac_V1/3(Vf)  "Vfd"
  Steam Turbine and Governor1/4 -> DQN_Mac_V1/2(Pm)
  From12/1 -> abc to dq1/2  "theta"
  abc to dq1/1 -> Selector1/1  "vq,vd"
  Selector1/1 -> MATLAB Function1/1(Vdq_vec)
  From18/1 -> abc to dq1/1  "v"
  Clock/1 -> Gain12/1
  Gain12/1 -> [theta0]
  Gain/1 -> Demux6/1
  Step3/1 -> Steam Turbine and Governor1/2
  Constant1/1 -> Steam Turbine and Governor1/1
  DQN_Mac_V1/2(wm) -> Steam Turbine and Governor1/3
  DQN_Mac_V1/3(dtheta_e) -> Steam Turbine and Governor1/4
  [Vf] -> Mac_EMT/2
  From7/1 -> DQn->ABC/2(tho)  "theta"
  From16/1 -> Gain2/1
  From2/1 -> Mux/1  "Iabc_B22 (A)"
  From4/1 -> Mux/2  "v"
  Mux4/1 -> XY3/1
  Mux5/1 -> XY3/2
  From9/1 -> Mux4/1  "Vabc_EMT"
  From8/1 -> Gain1/1  "Iabc_B22 (A)"
  Demux/2 -> Mux5/2  "Iabc_SS"
  Demux/1 -> Mux4/2  "Vabc_SS"
  Gain1/1 -> Mux5/1  "Iabc_EMT"
  Demux_DQNc_Mat2/1 -> DQn->ABC1/1(Xdcpnz_c), DQN_Mac_V1/1(Vs_C)  "[N+1,18 (6+6+6)]"
  Gain2/1 -> MatMux1/1(In1)
  Step1/1 -> [Pref]
  From11/1 -> DQn->ABC1/2(tho)  "theta"
  From15/1 -> DQn->ABC2/2(tho)  "theta"
  Demux_DQNc_Mat2/2 -> DQn->ABC2/1(Xdcpnz_c)  "[N+1,18 (6+6+6)]"
  DQn->ABC2/1(Xabc) -> Mux5/3  "Iabc_DQN"
  DQn->ABC1/1(Xabc) -> Mux4/3  "Vabc_DQN"
  Mux/1 -> State-Space/1
  State-Space/1 -> Demux/1
  [Vabc_BSRC] -> Mux6/2  "v"
  [Iabc_B222] -> Mux6/1  "Iabc_B22 (A)"
  SS_discrete/1(Y) -> Demux1/1
  Mux6/1 -> SS_discrete/1(U)
  Mux7/1 -> XY1/1
  Mux8/1 -> XY1/2
  Demux1/1 -> Mux7/2  "Vabc_SS"
  Demux1/2 -> Mux8/2  "Iabc_SS"
  Mux9/1 -> State-Space1/1
  State-Space1/1 -> Demux2/1
  Demux2/2 -> ?  "Iabc_SS"
  [Vabc_BSRC] -> Mux9/2  "v"
  [Iabc_B222] -> Mux9/1  "Iabc_B22 (A)"
  Demux2/1 -> Mux7/1  "Vabc_SS"
  connections:
  RL_src/RConn2 -- B500/RConn2
  B500/RConn1 -- RL_src/RConn1
  RL_src/RConn3 -- B500/RConn3
  B22/LConn1 -- Mac_EMT/RConn1 -- Load Flow Bus/LConn1
  ParallelRLC22/LConn1 -- B500/LConn1 -- B22/RConn1
  B22/RConn2 -- B500/LConn2 -- ParallelRLC22/LConn2
  ParallelRLC22/LConn3 -- B500/LConn3 -- B22/RConn3
  B1/LConn1 -- RL_src/LConn1
  Ground/LConn1 -- ParallelRLC22/RConn2 -- ParallelRLC22/RConn3 -- ParallelRLC22/RConn1
  RL_src/LConn2 -- B1/LConn2
  RL_src/LConn3 -- B1/LConn3
  B1/RConn1 -- Load Flow Bus1/LConn1 -- 500 kV 3333 MVA/RConn1
  B1/RConn2 -- 500 kV 3333 MVA/RConn2
  B1/RConn3 -- 500 kV 3333 MVA/RConn3
  Mac_EMT/RConn3 -- B22/LConn3
  Mac_EMT/RConn2 -- B22/LConn2

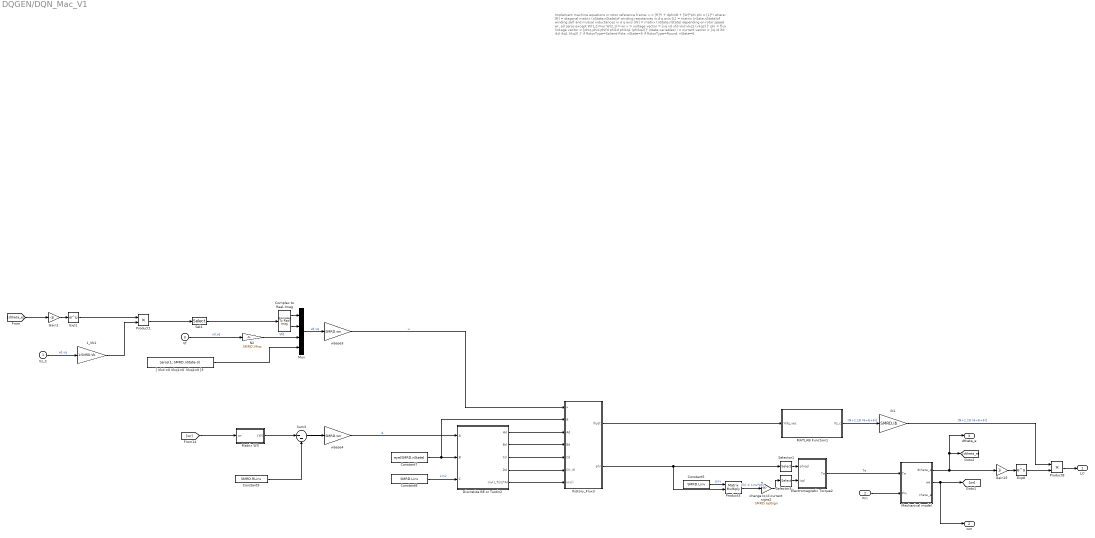
== system DQGEN/DQN_Mac_V1 ==
  note: Implement  machine equations in rotor reference frame:
      |   v = [R]*i + dphi/dt + [W]*phi
      | phi = [L]*i
      |
      | where:
      | [R] = diagonal matrix (nState,nState)of winding resistances in d q axis
      | [L] = matrix (nSate,nState)of winding self and mutual inductances in d q axis
      | [W] = matrix (nState,nState) depending on rotor speed wr,
      |       all zeros except W(1,2)=wr  W(2,1)=-wr
      |
      |   v = voltage vector      = [vq   vd   vfd   vkd   vkq1   (vkq2)  ]'
      | phi = flux linkage vector = [phiq phid phifd phikd phikq1 (phikq2)]' (state variables)
      |   i = current vector      = [iq   id   ifd   ikd   ikq1   (ikq2)  ]'
      |
      | if RotorType=Salient-Pole, nState=5
      | if RotorType=Round,        nState=6
  Vs_C : Inport
  Pm : Inport  Port=2
  Vf : Inport  Port=3
  1_Vb1 : Gain  Gain=1/SMRD.Vb  SaturateOnIntegerOverflow=on  OutDataTypeStr=Inherit: Same as input  ParamDataTypeStr=Inherit: Same as input
  Complex to Real-Imag : ComplexToRealImag
  Constant5 : Constant  Value=SMRD.Linv
  Constant7 : Constant  Value=eye(SMRD.nState)
  Constant8 : Constant  Value=SMRD.Linv
  Constant9 : Constant  Value=SMRD.RLinv
  Discretize BE or Tustin2 : Subsystem  AncestorBlock="spsSynchronousMachineModel/Discrete robust/State Space Model/Discretize  BE or Tustin"
  Electromagnetic Torque2 : Subsystem
  Exp1 : Math
  Exp8 : Math
  Gain1 : Gain  Gain=-1i
  Gain15 : Gain  Gain=1i
  Ihistory_Flux3 : Subsystem  AncestorBlock=spsSynchronousMachineModel/Discrete robust/State Space Model/Ihistory_Flux
  MATLAB Function1 : MATLAB Function  TreatAsAtomicUnit=on  mask{N=SMRD.N}
      mask prompts: N "Harmonic order:"
  Matrix W3 : Subsystem
  Mechanical model : Subsystem
      settings: LibrarySourceBlock=spsSynchronousMachineModel/Discrete Pm input trapezoidal
  Mux : Mux
  N2 : Gain  Gain=SMRD.Vfnp  SaturateOnIntegerOverflow=on  OutDataTypeStr=Inherit: Same as input  ParamDataTypeStr=Inherit: Same as input
  Product1 : Product
  Product3 : Product  Multiplication=Matrix(*)  SaturateOnIntegerOverflow=on  OutDataTypeStr=Inherit: Same as first input
  Product8 : Product
  Sel4 : Selector  NumberOfDimensions=2  InputPortWidth=3  IndexOptions=Index vector (dialog),Index vector (dialog)  Indices=1,2  OutputSizes=1
  Selector1 : Selector  InputPortWidth=SMRD.nState  IndexOptions=Index vector (dialog)  Indices=[1 2]  OutputSizes=1
  Selector3 : Selector  InputPortWidth=SMRD.nState  IndexOptions=Index vector (dialog)  Indices=[1 2]  OutputSizes=1
  Sum3 : Sum  Inputs=|--  SaturateOnIntegerOverflow=on
  "[ Vkd =0 Vkq1=0  Vkq2=0 ]3" : Constant  Value=zeros(1, SMRD.nState-3)
  change Iq Id current signs2 : Gain  Gain=SMRD.IqdSign
  ib1 : Gain  Gain=SMRD.Ib  SaturateOnIntegerOverflow=on  OutDataTypeStr=Inherit: Same as input  ParamDataTypeStr=Inherit: Same as input
  wbase3 : Gain  Gain=SMRD.wn  SaturateOnIntegerOverflow=on  OutDataTypeStr=Inherit: Same as input  ParamDataTypeStr=Inherit: Same as input
  wbase4 : Gain  Gain=SMRD.wn  SaturateOnIntegerOverflow=on  OutDataTypeStr=Inherit: Same as input  ParamDataTypeStr=Inherit: Same as input
  I_C : Outport  VectorParamsAs1DForOutWhenUnconnected=off
  wm : Outport  Port=2  VectorParamsAs1DForOutWhenUnconnected=off
  dtheta_e : Outport  Port=3  VectorParamsAs1DForOutWhenUnconnected=off
  wires:
  [dtheta_e] -> Gain1/1
  Mechanical model/1(dtheta_e) -> Gain15/1, dtheta_e/1, [dtheta_e]
  Product1/1 -> Sel4/1
  Exp1/1 -> Product1/1
  Gain1/1 -> Exp1/1
  Exp8/1 -> Product8/2
  Product8/1 -> I_C/1
  Gain15/1 -> Exp8/1
  Ihistory_Flux3/2(phi) -> Product3/2, Selector1/1
  wbase4/1 -> Discretize BE or Tustin2/1(A)  "A"
  Constant9/1 -> Sum3/2
  Matrix W3/1("[W]") -> Sum3/1
  [wr] -> Matrix W3/1(wr)
  Constant8/1 -> Discretize BE or Tustin2/3(C)  "Linv"
  Ihistory_Flux3/1(Ihyst) -> MATLAB Function1/1(Vdq_vec)
  Sum3/1 -> wbase4/1
  Constant7/1 -> Discretize BE or Tustin2/2(B), Ihistory_Flux3/2(B)
  Discretize BE or Tustin2/3(Cd) -> Ihistory_Flux3/5(Cd)
  Discretize BE or Tustin2/2(Bd) -> Ihistory_Flux3/4(Bd)
  Discretize BE or Tustin2/1(Ad) -> Ihistory_Flux3/3(Ad)
  Discretize BE or Tustin2/5(inv(I_Ts/2*A)) -> Ihistory_Flux3/7(inv())
  Discretize BE or Tustin2/4(Dd) -> Ihistory_Flux3/6(D(:,3))
  wbase3/1 -> Ihistory_Flux3/1(u)  "u"
  "[ Vkd =0 Vkq1=0  Vkq2=0 ]3"/1 -> Mux/4
  1_Vb1/1 -> Product1/2
  Vf/1 -> N2/1  "vd,vq"
  Vs_C/1 -> 1_Vb1/1  "vd,vq"
  Mechanical model/2(we) -> wm/1, [wr]
  Mux/1 -> wbase3/1  "vd,vq"
  N2/1 -> Mux/3  "Vfd"
  Complex to Real-Imag/1 -> Mux/1
  Complex to Real-Imag/2 -> Mux/2
  Sel4/1 -> Complex to Real-Imag/1
  ib1/1 -> Product8/1  "[N+1,18 (6+6+6)]"
  MATLAB Function1/1(Vs_c) -> ib1/1  "[N+1,18 (6+6+6)]"
  change Iq Id current signs2/1 -> Selector3/1
  Electromagnetic Torque2/1(Te) -> Mechanical model/1(Te)  "Te"
  Pm/1 -> Mechanical model/2(Pm)
  Product3/1 -> change Iq Id current signs2/1  "I(k) = Linv*phi"
  Selector1/1 -> Electromagnetic Torque2/1(phiqd)
  Constant5/1 -> Product3/1  "Linv"
  Selector3/1 -> Electromagnetic Torque2/2(iqd)

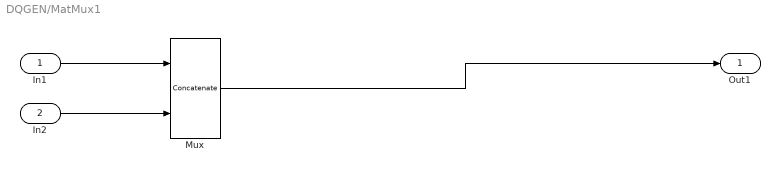
== system DQGEN/MatMux1 ==
  In1 : Inport
  In2 : Inport  Port=2
  Mux : Concatenate  Mode=Multidimensional array
  Out1 : Outport
  wires:
  In1/1 -> Mux/1
  In2/1 -> Mux/2
  Mux/1 -> Out1/1

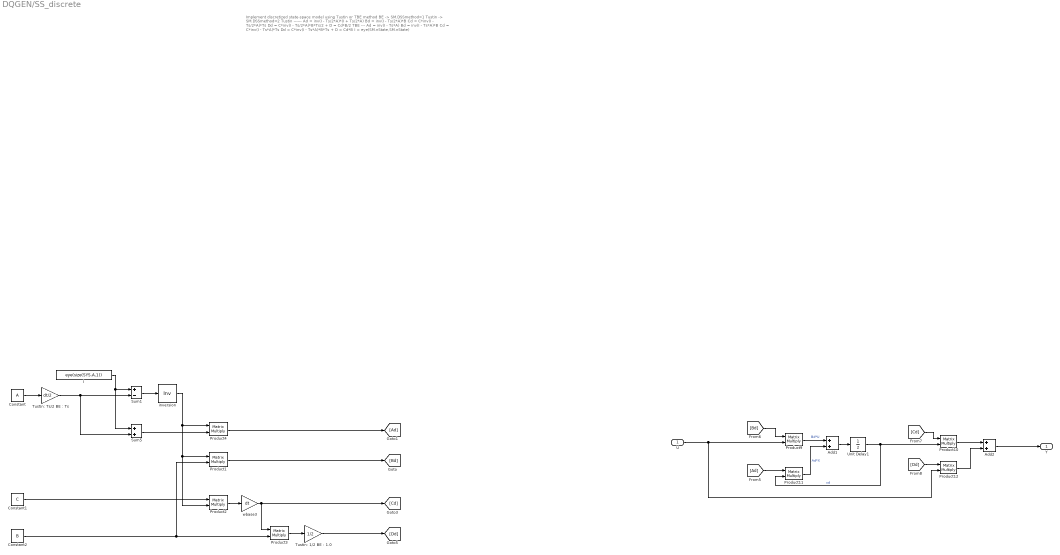
== system DQGEN/SS_discrete ==
  note: Implement discretized state-space model using Tustin or TBE method
      |
      | BE      -> SM.DSSmethod=1
      | Tustin  -> SM.DSSmethod=2
      |
      |
      | Tustin
      | ------
      | Ad = inv(I - Ts/2*A)*(I + Ts/2*A)
      | Bd = inv(I - Ts/2*A)*B
      | Cd = C*inv(I - Ts/2*A)*Ts
      | Dd = C*inv(I - Ts/2*A)*B*Ts/2  + D  =  Cd*B/2
      |
      | TBE
      | ---
      | Ad = inv(I - Ts*A)
      | Bd = inv(I - Ts*A)*B
      | Cd = C*inv(I - Ts*A)*Ts
      | Dd = C*inv(I - Ts*A)*B*Ts  + D  =  Cd*B
      |
      | I = eye(SM.nState,SM.nState)
  U : Inport
  Add1 : Sum
  Add2 : Sum
  Constant : Constant  Value=A
  Constant1 : Constant  Value=C
  Constant2 : Constant  Value=B
  I : Constant  Value=eye(size(SYS.A,1))
  Product{1..4,9..12} (8 alike) : Product  Multiplication=Matrix(*)  SaturateOnIntegerOverflow=on  OutDataTypeStr=Inherit: Same as first input
  Sum1 : Sum  Inputs=+-  SaturateOnIntegerOverflow=on
  Sum5 : Sum  SaturateOnIntegerOverflow=on
  "Tustin: 1/2 BE : 1.0" : Gain  Gain=1/2  SaturateOnIntegerOverflow=on  OutDataTypeStr=Inherit: Same as input  ParamDataTypeStr=Inherit: Same as input
  "Tustin: Ts/2 BE : Ts" : Gain  Gain=dt/2  SaturateOnIntegerOverflow=on  OutDataTypeStr=Inherit: Same as input  ParamDataTypeStr=Inherit: Same as input
  Unit Delay1 : UnitDelay  SampleTime=dt  HasFrameUpgradeWarning=on
  inversion : Product  Inputs=/  Multiplication=Matrix(*)  RndMeth=Zero
  wbase3 : Gain  Gain=dt  SaturateOnIntegerOverflow=on  OutDataTypeStr=Inherit: Same as input  ParamDataTypeStr=Inherit: Same as input
  Y : Outport
  wires:
  Product12/1 -> Add2/2
  [Ad] -> Product11/1
  [Dd] -> Product12/1
  Product10/1 -> Add2/1
  [Bd] -> Product9/1
  Unit Delay1/1 -> Product11/2, Product10/2  "xd"
  [Cd] -> Product10/1
  Product9/1 -> Add1/1  "Bd*U"
  Add1/1 -> Unit Delay1/1
  Product11/1 -> Add1/2  "Ad*X"
  U/1 -> Product12/2, Product9/2
  wbase3/1 -> [Cd], Product3/1
  "Tustin: 1/2 BE : 1.0"/1 -> [Dd]
  Constant1/1 -> Product2/1
  Product1/1 -> [Bd]
  Constant2/1 -> Product1/2, Product3/2
  Sum5/1 -> Product4/2
  Product3/1 -> "Tustin: 1/2 BE : 1.0"/1
  "Tustin: Ts/2 BE : Ts"/1 -> Sum5/2, Sum1/2
  Product2/1 -> wbase3/1
  Sum1/1 -> inversion/1
  Constant/1 -> "Tustin: Ts/2 BE : Ts"/1
  inversion/1 -> Product2/2, Product1/1, Product4/1
  I/1 -> Sum5/1, Sum1/1
  Product4/1 -> [Ad]
  Add2/1 -> Y/1

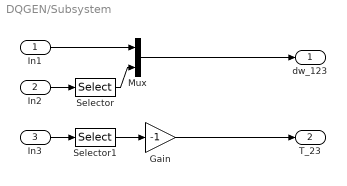
== system DQGEN/Subsystem ==
  In1 : Inport
  In2 : Inport  Port=2
  In3 : Inport  Port=3
  Gain : Gain  Gain=-1  SaturateOnIntegerOverflow=on  OutDataTypeStr=Inherit: Same as input  ParamDataTypeStr=Inherit: Same as input
  Mux : Mux  Inputs=2
  Selector : Selector  InputPortWidth=4  IndexOptions=Index vector (dialog)  Indices=[4 3]  OutputSizes=1
  Selector1 : Selector  InputPortWidth=4  IndexOptions=Index vector (dialog)  Indices=[4 3]  OutputSizes=1
  dw_123 : Outport  VectorParamsAs1DForOutWhenUnconnected=off
  T_23 : Outport  Port=2  VectorParamsAs1DForOutWhenUnconnected=off
  wires:
  Selector/1 -> Mux/2
  Mux/1 -> dw_123/1
  In1/1 -> Mux/1
  In2/1 -> Selector/1
  In3/1 -> Selector1/1
  Selector1/1 -> Gain/1
  Gain/1 -> T_23/1

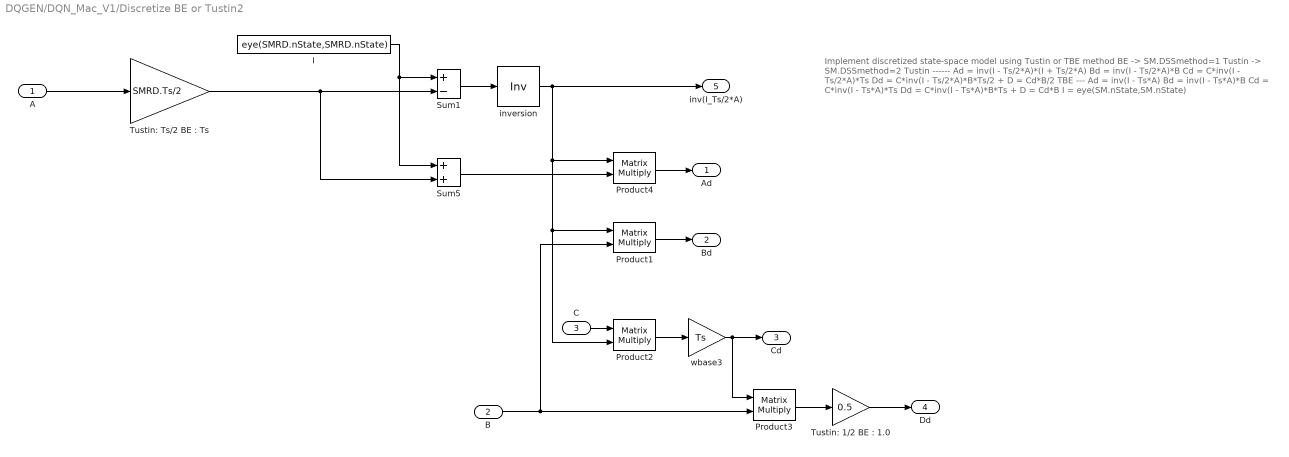
== system DQGEN/DQN_Mac_V1/Discretize BE or Tustin2 ==
  note: Implement discretized state-space model using Tustin or TBE method
      |
      | BE      -> SM.DSSmethod=1
      | Tustin  -> SM.DSSmethod=2
      |
      |
      | Tustin
      | ------
      | Ad = inv(I - Ts/2*A)*(I + Ts/2*A)
      | Bd = inv(I - Ts/2*A)*B
      | Cd = C*inv(I - Ts/2*A)*Ts
      | Dd = C*inv(I - Ts/2*A)*B*Ts/2  + D  =  Cd*B/2
      |
      | TBE
      | ---
      | Ad = inv(I - Ts*A)
      | Bd = inv(I - Ts*A)*B
      | Cd = C*inv(I - Ts*A)*Ts
      | Dd = C*inv(I - Ts*A)*B*Ts  + D  =  Cd*B
      |
      | I = eye(SM.nState,SM.nState)
  A : Inport
  B : Inport  Port=2
  C : Inport  Port=3
  I : Constant  Value=eye(SMRD.nState,SMRD.nState)
  Product{1..4} (4 alike) : Product  Multiplication=Matrix(*)  SaturateOnIntegerOverflow=on  OutDataTypeStr=Inherit: Same as first input
  Sum1 : Sum  Inputs=+-  SaturateOnIntegerOverflow=on
  Sum5 : Sum  SaturateOnIntegerOverflow=on
  "Tustin: 1/2 BE : 1.0" : Gain  Gain=0.5  SaturateOnIntegerOverflow=on  OutDataTypeStr=Inherit: Same as input  ParamDataTypeStr=Inherit: Same as input
  "Tustin: Ts/2 BE : Ts" : Gain  Gain=SMRD.Ts/2  SaturateOnIntegerOverflow=on  OutDataTypeStr=Inherit: Same as input  ParamDataTypeStr=Inherit: Same as input
  inversion : Product  Inputs=/  Multiplication=Matrix(*)  RndMeth=Zero
  wbase3 : Gain  Gain=Ts  SaturateOnIntegerOverflow=on  OutDataTypeStr=Inherit: Same as input  ParamDataTypeStr=Inherit: Same as input
  Ad : Outport  VectorParamsAs1DForOutWhenUnconnected=off
  Bd : Outport  Port=2  VectorParamsAs1DForOutWhenUnconnected=off
  Cd : Outport  Port=3  VectorParamsAs1DForOutWhenUnconnected=off
  Dd : Outport  Port=4  VectorParamsAs1DForOutWhenUnconnected=off
  inv(I_Ts/2*A) : Outport  Port=5  VectorParamsAs1DForOutWhenUnconnected=off
  wires:
  wbase3/1 -> Product3/1, Cd/1
  "Tustin: 1/2 BE : 1.0"/1 -> Dd/1
  Product3/1 -> "Tustin: 1/2 BE : 1.0"/1
  Product2/1 -> wbase3/1
  C/1 -> Product2/1
  B/1 -> Product3/2, Product1/2
  Product1/1 -> Bd/1
  Sum5/1 -> Product4/2
  inversion/1 -> inv(I_Ts/2*A)/1, Product4/1, Product1/1, Product2/2
  Sum1/1 -> inversion/1
  I/1 -> Sum1/1, Sum5/1
  A/1 -> "Tustin: Ts/2 BE : Ts"/1
  Product4/1 -> Ad/1
  "Tustin: Ts/2 BE : Ts"/1 -> Sum5/2, Sum1/2

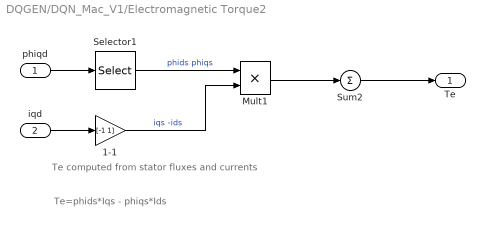
== system DQGEN/DQN_Mac_V1/Electromagnetic Torque2 ==
  note: Te=phids*Iqs - phiqs*Ids
  note: Te computed from stator fluxes and currents
  phiqd : Inport
  iqd : Inport  Port=2
  1-1 : Gain  Gain=[-1 1]
  Mult1 : Product  Inputs=**
  Selector1 : Selector  InputPortWidth=2  IndexOptions=Index vector (dialog)  Indices="[2  1]"  OutputSizes=1
  Sum2 : Sum  Inputs=1  SaturateOnIntegerOverflow=on
  Te : Outport  VectorParamsAs1DForOutWhenUnconnected=off
  wires:
  Sum2/1 -> Te/1
  Selector1/1 -> Mult1/1  "phids phiqs"
  1-1/1 -> Mult1/2  "iqs -ids"
  iqd/1 -> 1-1/1
  Mult1/1 -> Sum2/1
  phiqd/1 -> Selector1/1

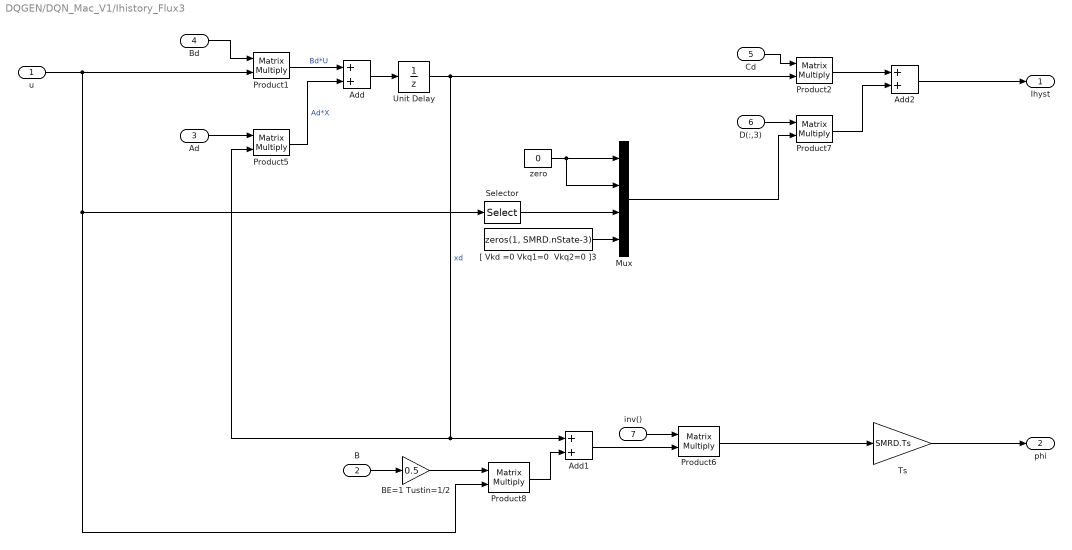
== system DQGEN/DQN_Mac_V1/Ihistory_Flux3 ==
  u : Inport
  B : Inport  Port=2
  Ad : Inport  Port=3
  Bd : Inport  Port=4
  Cd : Inport  Port=5
  D(:,3) : Inport  Port=6
  inv() : Inport  Port=7
  Add : Sum
  Add1 : Sum
  Add2 : Sum
  BE=1 Tustin=1/2 : Gain  Gain=0.5
  Mux : Mux
  Product{1..2,5..8} (6 alike) : Product  Multiplication=Matrix(*)  SaturateOnIntegerOverflow=on  OutDataTypeStr=Inherit: Same as first input
  Selector : Selector  InputPortWidth=SMRD.nState  IndexOptions=Index vector (dialog)  Indices=[3]  OutputSizes=1
  Ts : Gain  Gain=SMRD.Ts  SaturateOnIntegerOverflow=on  OutDataTypeStr=Inherit: Same as input  ParamDataTypeStr=Inherit: Same as input
  Unit Delay : UnitDelay  InitialCondition=SMRD.phidq0(1:SMRD.nState)/SMRD.Ts  SampleTime=SMRD.Ts  HasFrameUpgradeWarning=on
  "[ Vkd =0 Vkq1=0  Vkq2=0 ]3" : Constant  Value=zeros(1, SMRD.nState-3)
  zero : Constant  Value=0
  Ihyst : Outport  VectorParamsAs1DForOutWhenUnconnected=off
  phi : Outport  Port=2  VectorParamsAs1DForOutWhenUnconnected=off
  wires:
  Product7/1 -> Add2/2
  Selector/1 -> Mux/3
  zero/1 -> Mux/1, Mux/2
  "[ Vkd =0 Vkq1=0  Vkq2=0 ]3"/1 -> Mux/4
  D(:,3)/1 -> Product7/1
  Mux/1 -> Product7/2
  Add2/1 -> Ihyst/1
  Product2/1 -> Add2/1
  Ts/1 -> phi/1
  Product1/1 -> Add/1  "Bd*U"
  Add/1 -> Unit Delay/1
  Unit Delay/1 -> Product2/2, Add1/1, Product5/2  "xd"
  Product5/1 -> Add/2  "Ad*X"
  Product6/1 -> Ts/1
  Product8/1 -> Add1/2
  Add1/1 -> Product6/2
  Ad/1 -> Product5/1
  Bd/1 -> Product1/1
  Cd/1 -> Product2/1
  inv()/1 -> Product6/1
  B/1 -> BE=1 Tustin=1/2/1
  u/1 -> Selector/1, Product8/2, Product1/2
  BE=1 Tustin=1/2/1 -> Product8/1

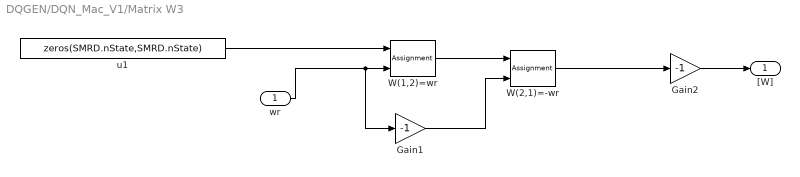
== system DQGEN/DQN_Mac_V1/Matrix W3 ==
  wr : Inport
  Gain1 : Gain  Gain=-1  SaturateOnIntegerOverflow=on  OutDataTypeStr=Inherit: Same as input  ParamDataTypeStr=Inherit: Same as input
  Gain2 : Gain  Gain=-1  SaturateOnIntegerOverflow=on  OutDataTypeStr=Inherit: Same as input  ParamDataTypeStr=Inherit: Same as input
  W(1,2)=wr : Assignment  NumberOfDimensions=2  IndexOptions=Index vector (dialog),Index vector (dialog)  Indices=1,2  OutputSizes=1,1
  W(2,1)=-wr : Assignment  NumberOfDimensions=2  IndexOptions=Index vector (dialog),Index vector (dialog)  Indices=2,1  OutputSizes=1,1
  u1 : Constant  Value=zeros(SMRD.nState,SMRD.nState)
  "[W]" : Outport  VectorParamsAs1DForOutWhenUnconnected=off
  wires:
  Gain2/1 -> "[W]"/1
  W(2,1)=-wr/1 -> Gain2/1
  wr/1 -> Gain1/1, W(1,2)=wr/2
  W(1,2)=wr/1 -> W(2,1)=-wr/1
  Gain1/1 -> W(2,1)=-wr/2
  u1/1 -> W(1,2)=wr/1

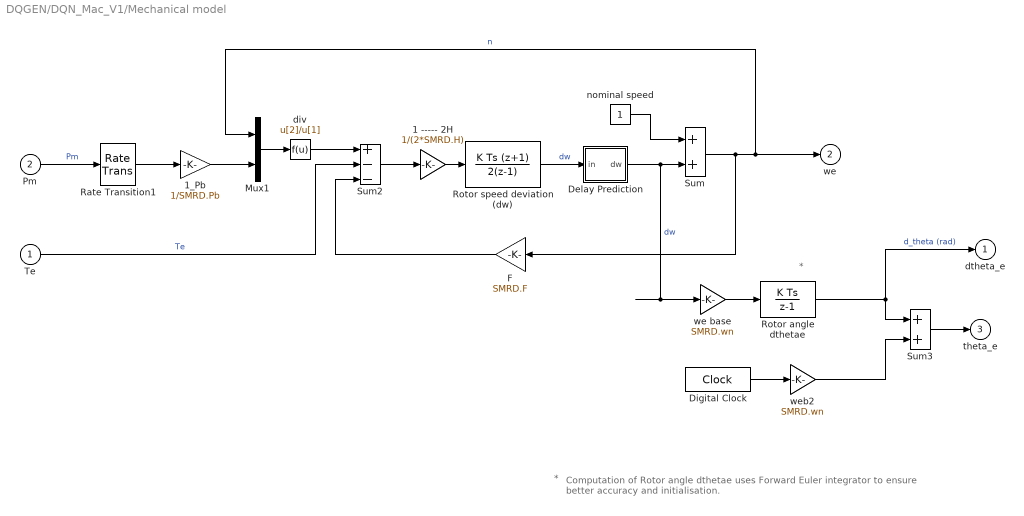
== system DQGEN/DQN_Mac_V1/Mechanical model ==
  note: *
  note: Computation of Rotor angle dthetae uses Forward Euler
      | integrator to ensure better accuracy and initialisation.
  note: *
  Te : Inport  PortDimensions=1
  Pm : Inport  Port=2
  1 ----- 2H : Gain  Gain=1/(2*SMRD.H)  SaturateOnIntegerOverflow=on  OutDataTypeStr=Inherit: Same as input  ParamDataTypeStr=Inherit: Same as input
  1_Pb : Gain  Gain=1/SMRD.Pb  SaturateOnIntegerOverflow=on  OutDataTypeStr=Inherit: Same as input  ParamDataTypeStr=Inherit: Same as input
  Delay Prediction : Subsystem
  Digital Clock : DigitalClock  SampleTime=Ts
  F : Gain  Gain=SMRD.F  SaturateOnIntegerOverflow=on  OutDataTypeStr=Inherit: Same as input  ParamDataTypeStr=Inherit: Same as input
  Mux1 : Mux  Inputs=2
  Rate Transition1 : RateTransition  Deterministic=off  OutPortSampleTime=Ts
  Rotor angle dthetae : DiscreteIntegrator  InitialCondition=SMRD.tho  SampleTime=SMRD.Ts  ICPrevOutput=DiscIntNeverNeededParam  ICPrevScaledInput=DiscIntNeverNeededParam
  Rotor speed deviation (dw) : DiscreteIntegrator  IntegratorMethod=Integration: Trapezoidal  InitialCondition=SMRD.dwo  SampleTime=SMRD.Ts  ICPrevOutput=DiscIntNeverNeededParam  ICPrevScaledInput=DiscIntNeverNeededParam
  Sum : Sum  InputSameDT=on  SaturateOnIntegerOverflow=on  OutDataTypeStr=Inherit: Same as first input
  Sum2 : Sum  Inputs=+--  InputSameDT=on  SaturateOnIntegerOverflow=on  OutDataTypeStr=Inherit: Same as first input
  Sum3 : Sum  InputSameDT=on  SaturateOnIntegerOverflow=on  OutDataTypeStr=Inherit: Same as first input
  div : Fcn  Expr=u[2]/u[1]
      mask Display: disp('/')
  nominal speed : Constant
  we base : Gain  Gain=SMRD.wn  SaturateOnIntegerOverflow=on  OutDataTypeStr=Inherit: Same as input  ParamDataTypeStr=Inherit: Same as input
  web2 : Gain  Gain=SMRD.wn  SaturateOnIntegerOverflow=on  OutDataTypeStr=Inherit: Same as input  ParamDataTypeStr=Inherit: Same as input
  dtheta_e : Outport  InitialOutput=0  VectorParamsAs1DForOutWhenUnconnected=off
  we : Outport  Port=2  InitialOutput=0  VectorParamsAs1DForOutWhenUnconnected=off
  theta_e : Outport  Port=3  InitialOutput=0  VectorParamsAs1DForOutWhenUnconnected=off
  wires:
  Sum3/1 -> theta_e/1
  Sum/1 -> Mux1/1, we/1, F/1  "n"
  Sum2/1 -> 1 ----- 2H/1
  F/1 -> Sum2/3
  1_Pb/1 -> Mux1/2
  Pm/1 -> Rate Transition1/1  "Pm"
  Mux1/1 -> div/1
  Te/1 -> Sum2/2  "Te"
  div/1 -> Sum2/1
  1 ----- 2H/1 -> Rotor speed deviation (dw)/1
  nominal speed/1 -> Sum/1
  Rotor speed deviation (dw)/1 -> Delay Prediction/1(in)  "dw"
  we base/1 -> Rotor angle dthetae/1
  Digital Clock/1 -> web2/1
  web2/1 -> Sum3/2
  Rotor angle dthetae/1 -> dtheta_e/1, Sum3/1  "d_theta (rad)"
  Rate Transition1/1 -> 1_Pb/1
  Delay Prediction/1(dw) -> Sum/2, we base/1  "dw"
